simulink subsystem "QuaternionUpdate"  (R2021a)
settings: Solver=VariableStepAuto  StartTime=0.0  StopTime=10.0  RelTol=1e-3
libraries: aerolibutil x1, sharedutil x1
settings Model: Creator=Laura  LastModifiedBy=Laura

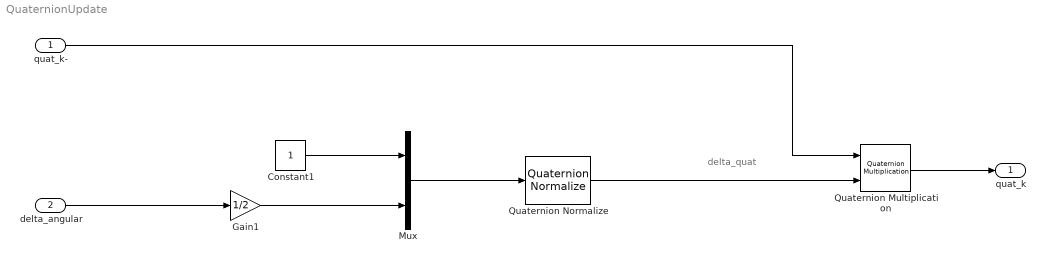
== system QuaternionUpdate ==
  note: delta_quat
  quat_k- : Inport  SampleTime=1/10
  delta_angular : Inport  Port=2  SampleTime=1/10
  Constant1 : Constant
  Gain1 : Gain  Gain=1/2
  Mux : Mux  Inputs=2
  Quaternion Multiplication : aerolibutil/Quaternion Multiplication
  Quaternion Normalize : sharedutil/Quaternion Normalize  aMode=aMode
      settings: SourceProductBaseCode=AE,PW,DR,MT,UV,VE
  quat_k : Outport  SampleTime=1/10
  wires:
  delta_angular/1 -> Gain1/1
  Gain1/1 -> Mux/2
  Constant1/1 -> Mux/1
  Quaternion Multiplication/1 -> quat_k/1
  quat_k-/1 -> Quaternion Multiplication/1
  Mux/1 -> Quaternion Normalize/1
  Quaternion Normalize/1 -> Quaternion Multiplication/2
